simulink library "CTRL_DSI"  (R2023b)
settings: Solver=VariableStepAuto  StartTime=0.0  StopTime=10.0  RelTol=1e-3
undefined symbols (not defined in the file or in its folder): CTRL_DSI_p_SwtTqDmdTot
libraries: CTRL_DSI_PedalRecalc x1, CTRL_DSI_MomentMethod x1, CTRL_DSI_PedalMap x1
settings Model: Creator=blatak  LastModifiedBy=blatak
settings ModelReferenceCC: EnableRefExpFcnMdlSchedulingChecks=on

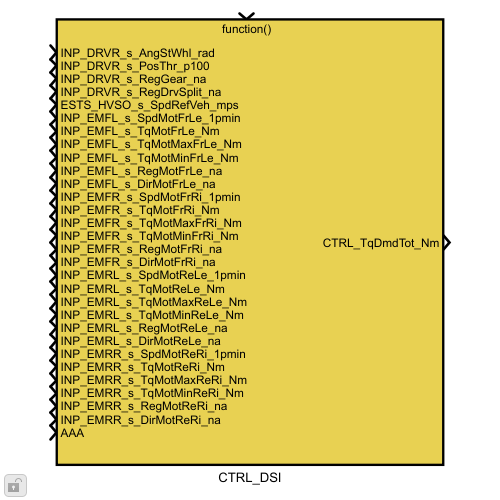
[thumbnail: Simulink's stored preview of the top-level diagram]
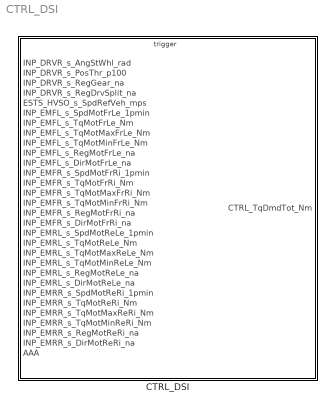
== system CTRL_DSI ==
  CTRL_DSI : Subsystem  TreatAsAtomicUnit=on

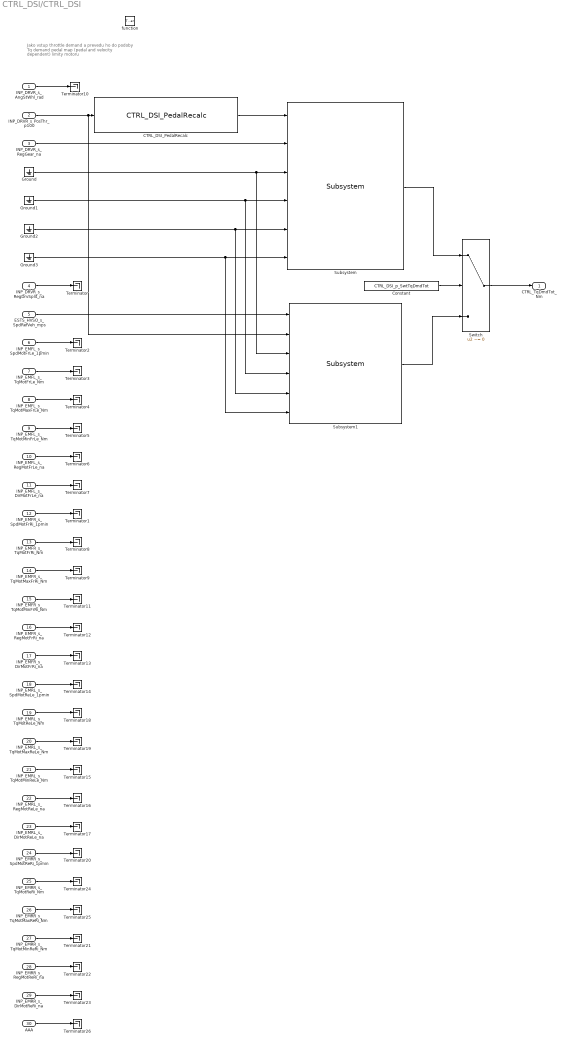
== system CTRL_DSI/CTRL_DSI ==
  note: Jako vstup throttle demand
      | a prevedu ho do podoby
      | Tq demand
      | pedal map (pedal and velocity dependent)
      | limity motoru
  INP_DRVR_s_AngStWhl_rad : Inport
  INP_DRVR_s_PosThr_p100 : Inport  Port=2
  INP_DRVR_s_RegGear_na : Inport  Port=3
  INP_DRVR_s_RegDrvSplit_na : Inport  Port=4
  ESTS_HVSO_s_SpdRefVeh_mps : Inport  Port=5
  INP_EMFL_s_SpdMotFrLe_1pmin : Inport  Port=6
  INP_EMFL_s_TqMotFrLe_Nm : Inport  Port=7
  INP_EMFL_s_TqMotMaxFrLe_Nm : Inport  Port=8
  INP_EMFL_s_TqMotMinFrLe_Nm : Inport  Port=9
  INP_EMFL_s_RegMotFrLe_na : Inport  Port=10
  INP_EMFL_s_DirMotFrLe_na : Inport  Port=11
  INP_EMFR_s_SpdMotFrRi_1pmin : Inport  Port=12
  INP_EMFR_s_TqMotFrRi_Nm : Inport  Port=13
  INP_EMFR_s_TqMotMaxFrRi_Nm : Inport  Port=14
  INP_EMFR_s_TqMotMinFrRi_Nm : Inport  Port=15
  INP_EMFR_s_RegMotFrRi_na : Inport  Port=16
  INP_EMFR_s_DirMotFrRi_na : Inport  Port=17
  INP_EMRL_s_SpdMotReLe_1pmin : Inport  Port=18
  INP_EMRL_s_TqMotReLe_Nm : Inport  Port=19
  INP_EMRL_s_TqMotMaxReLe_Nm : Inport  Port=20
  INP_EMRL_s_TqMotMinReLe_Nm : Inport  Port=21
  INP_EMRL_s_RegMotReLe_na : Inport  Port=22
  INP_EMRL_s_DirMotReLe_na : Inport  Port=23
  INP_EMRR_s_SpdMotReRi_1pmin : Inport  Port=24
  INP_EMRR_s_TqMotReRi_Nm : Inport  Port=25
  INP_EMRR_s_TqMotMaxReRi_Nm : Inport  Port=26
  INP_EMRR_s_TqMotMinReRi_Nm : Inport  Port=27
  INP_EMRR_s_RegMotReRi_na : Inport  Port=28
  INP_EMRR_s_DirMotReRi_na : Inport  Port=29
  AAA : Inport  Port=30
  function : TriggerPort  TriggerType=function-call  VariantControl=(inherit)
  CTRL_DSI_PedalRecalc : CTRL_DSI_PedalRecalc/CTRL_DSI_PedalRecalc  SystemSampleTime=-1  VariantActivationTime=update diagram  AllowFlexibleInterface=on  Latency=0  AutoFrameSizeCalculation=off
  Constant : Constant  Value=CTRL_DSI_p_SwtTqDmdTot
  Ground{,1..3} (4 alike) : Ground
  Subsystem : CTRL_DSI_MomentMethod/Subsystem  SystemSampleTime=-1  VariantActivationTime=update diagram  AllowFlexibleInterface=on  Latency=0  AutoFrameSizeCalculation=off
  Subsystem1 : CTRL_DSI_PedalMap/Subsystem  SystemSampleTime=-1  VariantActivationTime=update diagram  AllowFlexibleInterface=on  Latency=0  AutoFrameSizeCalculation=off
  Switch : Switch  Criteria=u2 ~= 0  SaturateOnIntegerOverflow=off  InputSameDT=off
  Terminator{,1..26} (27 alike) : Terminator
  CTRL_TqDmdTot_Nm : Outport
  wires:
  INP_DRVR_s_PosThr_p100/1 -> Subsystem1/2, CTRL_DSI_PedalRecalc/1
  CTRL_DSI_PedalRecalc/1 -> Subsystem/1
  INP_DRVR_s_RegGear_na/1 -> Subsystem/2
  Ground/1 -> Subsystem1/3, Subsystem/3
  Ground1/1 -> Subsystem1/4, Subsystem/4
  Ground3/1 -> Subsystem1/6, Subsystem/6
  Ground2/1 -> Subsystem1/5, Subsystem/5
  INP_DRVR_s_RegDrvSplit_na/1 -> Terminator/1
  ESTS_HVSO_s_SpdRefVeh_mps/1 -> Subsystem1/1
  INP_EMFL_s_SpdMotFrLe_1pmin/1 -> Terminator2/1
  INP_EMFL_s_TqMotFrLe_Nm/1 -> Terminator3/1
  INP_EMFL_s_TqMotMaxFrLe_Nm/1 -> Terminator4/1
  INP_EMFL_s_TqMotMinFrLe_Nm/1 -> Terminator5/1
  INP_EMFL_s_RegMotFrLe_na/1 -> Terminator6/1
  Switch/1 -> CTRL_TqDmdTot_Nm/1
  Constant/1 -> Switch/2
  Subsystem/1 -> Switch/1
  INP_DRVR_s_AngStWhl_rad/1 -> Terminator10/1
  Subsystem1/1 -> Switch/3
  INP_EMFL_s_DirMotFrLe_na/1 -> Terminator7/1
  INP_EMFR_s_RegMotFrRi_na/1 -> Terminator12/1
  INP_EMFR_s_TqMotMinFrRi_Nm/1 -> Terminator11/1
  INP_EMFR_s_TqMotMaxFrRi_Nm/1 -> Terminator9/1
  INP_EMFR_s_SpdMotFrRi_1pmin/1 -> Terminator1/1
  INP_EMFR_s_TqMotFrRi_Nm/1 -> Terminator8/1
  INP_EMFR_s_DirMotFrRi_na/1 -> Terminator13/1
  INP_EMRL_s_DirMotReLe_na/1 -> Terminator17/1
  INP_EMRL_s_TqMotMinReLe_Nm/1 -> Terminator15/1
  INP_EMRL_s_SpdMotReLe_1pmin/1 -> Terminator14/1
  INP_EMRL_s_RegMotReLe_na/1 -> Terminator16/1
  INP_EMRL_s_TqMotMaxReLe_Nm/1 -> Terminator19/1
  INP_EMRL_s_TqMotReLe_Nm/1 -> Terminator18/1
  INP_EMRR_s_DirMotReRi_na/1 -> Terminator23/1
  INP_EMRR_s_TqMotMaxReRi_Nm/1 -> Terminator25/1
  INP_EMRR_s_SpdMotReRi_1pmin/1 -> Terminator20/1
  INP_EMRR_s_TqMotMinReRi_Nm/1 -> Terminator21/1
  INP_EMRR_s_RegMotReRi_na/1 -> Terminator22/1
  INP_EMRR_s_TqMotReRi_Nm/1 -> Terminator24/1
  AAA/1 -> Terminator26/1
